simulink model "Q2"  (R2021a)
settings: Solver=VariableStepAuto  StartTime=0.0  StopTime=16000  RelTol=1e-3
settings Model: Creator=viral  LastModifiedBy=viral

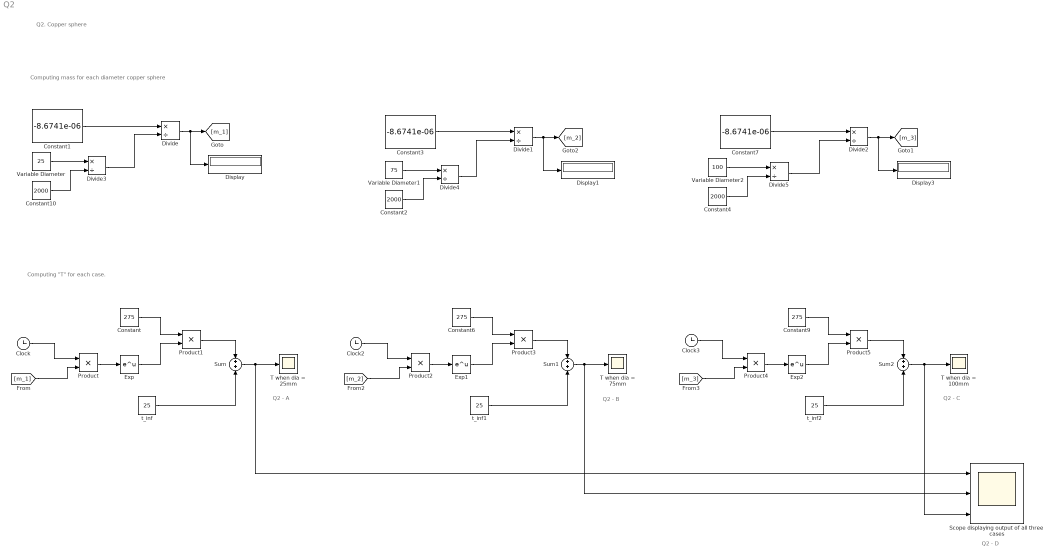
== system Q2 ==
  note: Computing mass for each diameter copper sphere
  note: Computing "T" for each case.
  note: Q2. Copper sphere
  note: Q2 - A
  note: Q2 - B
  note: Q2 - C
  note: Q2 - D
  Clock : Clock
  Clock2 : Clock
  Clock3 : Clock
  Constant : Constant  Value=275
  Constant1 : Constant  Value=-8.6741e-06
  Constant10 : Constant  Value=2000
  Constant2 : Constant  Value=2000
  Constant3 : Constant  Value=-8.6741e-06
  Constant4 : Constant  Value=2000
  Constant6 : Constant  Value=275
  Constant7 : Constant  Value=-8.6741e-06
  Constant9 : Constant  Value=275
  Display : Display
  Display1 : Display
  Display3 : Display
  Divide{,1..5} (6 alike) : Product  Inputs=*/
  Exp : Math  SaturateOnIntegerOverflow=on
  Exp1 : Math  SaturateOnIntegerOverflow=on
  Exp2 : Math  SaturateOnIntegerOverflow=on
  Product{,1..5} (6 alike) : Product
  "Scope displaying output of all three cases " : Scope  NumInputPorts=3
  Sum : Sum  Inputs=+|+
  Sum1 : Sum  Inputs=+|+
  Sum2 : Sum  Inputs=+|+
  T when dia = 100mm : Scope
  T when dia = 25mm : Scope
  T when dia = 75mm : Scope
  Variable Diameter : Constant  Value=25
  Variable Diameter1 : Constant  Value=75
  Variable Diameter2 : Constant  Value=100
  t_inf : Constant  Value=25
  t_inf1 : Constant  Value=25
  t_inf2 : Constant  Value=25
  wires:
  Constant1/1 -> Divide/1
  Divide/1 -> Display/1, [m_1]
  [m_1] -> Product/2
  Product/1 -> Exp/1
  Constant/1 -> Product1/1
  Exp/1 -> Product1/2
  Product1/1 -> Sum/1
  t_inf/1 -> Sum/2
  Sum/1 -> "Scope displaying output of all three cases "/1, T when dia = 25mm/1
  Clock/1 -> Product/1
  Constant3/1 -> Divide1/1
  Divide1/1 -> Display1/1, [m_2]
  t_inf1/1 -> Sum1/2
  Product3/1 -> Sum1/1
  Clock2/1 -> Product2/1
  Sum1/1 -> "Scope displaying output of all three cases "/2, T when dia = 75mm/1
  Constant6/1 -> Product3/1
  [m_2] -> Product2/2
  Product2/1 -> Exp1/1
  Exp1/1 -> Product3/2
  Divide2/1 -> Display3/1, [m_3]
  Constant7/1 -> Divide2/1
  Sum2/1 -> "Scope displaying output of all three cases "/3, T when dia = 100mm/1
  t_inf2/1 -> Sum2/2
  Exp2/1 -> Product5/2
  Product4/1 -> Exp2/1
  Product5/1 -> Sum2/1
  [m_3] -> Product4/2
  Clock3/1 -> Product4/1
  Constant9/1 -> Product5/1
  Variable Diameter/1 -> Divide3/1
  Constant10/1 -> Divide3/2
  Divide3/1 -> Divide/2
  Constant2/1 -> Divide4/2
  Variable Diameter1/1 -> Divide4/1
  Divide4/1 -> Divide1/2
  Constant4/1 -> Divide5/2
  Variable Diameter2/1 -> Divide5/1
  Divide5/1 -> Divide2/2
